simulink model "test_cost_function_only_without_delays"  (R2022a)
settings: Solver=FixedStepDiscrete  StartTime=0.0  StopTime=10.0  RelTol=1e-3
undefined symbols (not defined in the file or in its folder): f_c
libraries: hdlsllib x1
settings Model: DataTypeOverride=Off  Creator=Andre Merx  LastModifiedBy=Andre Merx
settings SolverCC: AlgebraicLoopSolver=TrustRegion
settings DataIOCC: LimitDataPoints=on  SaveOutput=off  SaveTime=off
settings OptimizationCC: BlockReduction=off  ConditionallyExecuteInputs=off  DefaultParameterBehavior=Inlined  LifeSpan=inf
settings DebuggingCC: AlgebraicLoopMsg=error  SingleTaskRateTransMsg=error  UnconnectedInputMsg=warning  UnconnectedOutputMsg=warning  UnconnectedLineMsg=warning  AllowSymbolicDim=off  StrictBusMsg=ErrorOnBusTreatedAsVector  SFUnexpectedBacktrackingDiag=warning  SFNoUnconditionalDefaultTransitionDiag=warning  SFExecutionAtInitializationDiag=none  SFMachineParentedDataDiag=warning  ArithmeticOperatorsInVariantConditions=warning
settings HardwareCC: ProdBitPerPointer=32  ProdBitPerSizeT=32  ProdBitPerPtrDiffT=32  ProdLargestAtomicFloat=None  ProdIntDivRoundTo=Undefined  ProdEndianess=Unspecified  ProdWordSize=32  ProdHWDeviceType=ASIC/FPGA->ASIC/FPGA  ProdEqTarget=off
settings SFSimCC: SimUseLocalCustomCode=off  CustomCodeUndefinedFunction=UseInterfaceOnly
settings RTWCC: RTWUseLocalCustomCode=off
settings CodeAppCC: StateflowObjectComments=on
settings GRTTargetCC: TargetLangStandard=C89/C90 (ANSI)
settings ConfigComp: CovScope=ReferencedModels  CovMetricSettings=dw  CovSaveCumulativeToWorkspaceVar=on  CovSaveSingleToWorkspaceVar=on  CovExternalEMLEnable=off  CovSFcnEnable=off

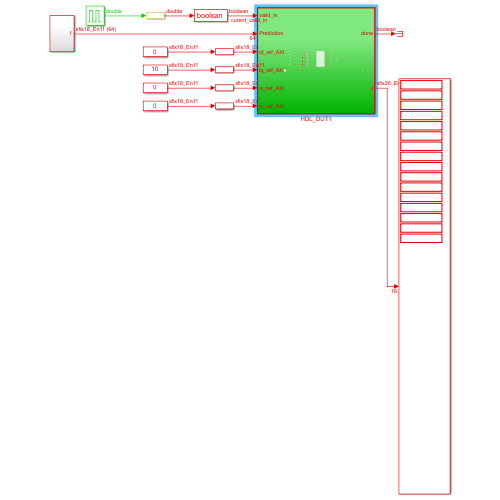
[thumbnail: Simulink's stored preview of the top-level diagram]
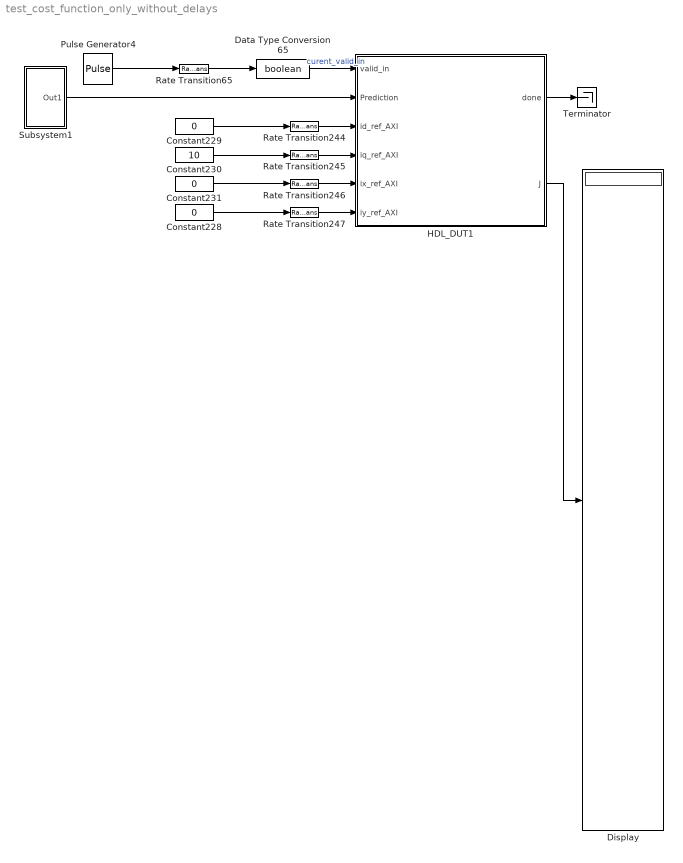
== system test_cost_function_only_without_delays ==
  Constant228 : Constant  Value=0  OutDataTypeStr=fixdt(1,18,11)  SampleTime=-1
  Constant229 : Constant  Value=0  OutDataTypeStr=fixdt(1,18,11)  SampleTime=-1
  Constant230 : Constant  Value=10  OutDataTypeStr=fixdt(1,18,11)  SampleTime=-1
  Constant231 : Constant  Value=0  OutDataTypeStr=fixdt(1,18,11)  SampleTime=-1
  Data Type Conversion65 : DataTypeConversion  OutDataTypeStr=boolean  SaturateOnIntegerOverflow=off  RndMeth=Floor
  Display : Display
  HDL_DUT1 : Subsystem  TreatAsAtomicUnit=on
  Pulse Generator4 : DiscretePulseGenerator  PulseType=Time based  Period=1/f_c
  Rate Transition{65,244..247} (5 alike) : RateTransition  OutPortSampleTime=Rt
  Subsystem1 : Subsystem
  Terminator : Terminator
  wires:
  Constant228/1 -> Rate Transition247/1
  Constant231/1 -> Rate Transition246/1
  Rate Transition247/1 -> HDL_DUT1/6(iy_ref_AXI)
  Rate Transition245/1 -> HDL_DUT1/4(iq_ref_AXI)
  Subsystem1/1(Out1) -> HDL_DUT1/2(Prediction)
  Constant229/1 -> Rate Transition244/1
  Constant230/1 -> Rate Transition245/1
  Rate Transition246/1 -> HDL_DUT1/5(ix_ref_AXI)
  Rate Transition244/1 -> HDL_DUT1/3(id_ref_AXI)
  Pulse Generator4/1 -> Rate Transition65/1
  Rate Transition65/1 -> Data Type Conversion65/1
  Data Type Conversion65/1 -> HDL_DUT1/1(valid_in)  "curent_valid_in"
  HDL_DUT1/1(done) -> Terminator/1
  HDL_DUT1/2(J) -> Display/1

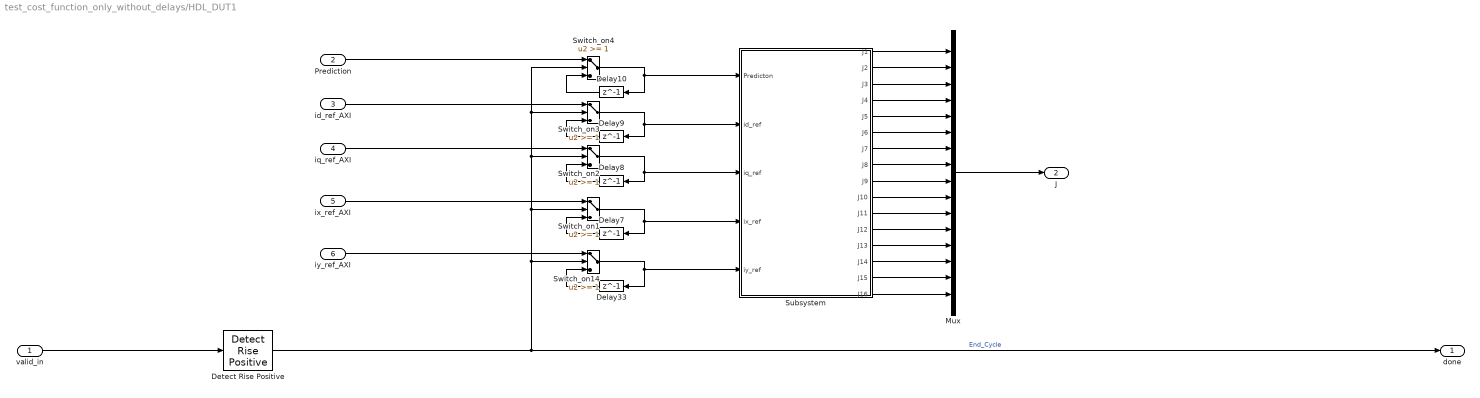
== system test_cost_function_only_without_delays/HDL_DUT1 ==
  valid_in : Inport
  Prediction : Inport  Port=2
  id_ref_AXI : Inport  Port=3
  iq_ref_AXI : Inport  Port=4
  ix_ref_AXI : Inport  Port=5
  iy_ref_AXI : Inport  Port=6
  Delay{7..10,33} (5 alike) : Delay  DelayLength=1
  Detect Rise Positive : hdlsllib/Logic and Bit Operations/Detect Rise Positive  vinit=0  OutDataTypeStr=boolean
      settings: SourceProductBaseCode=SL
  Mux : Mux  Inputs=16
  Subsystem : Subsystem
  Switch_on{1..4,14} (5 alike) : Switch  Threshold=1  OutDataTypeStr=fixdt(1,18,11)  RndMeth=Simplest  SaturateOnIntegerOverflow=off  InputSameDT=off
  done : Outport
  J : Outport  Port=2
  wires:
  iy_ref_AXI/1 -> Switch_on14/1
  Switch_on14/1 -> Delay33/1, Subsystem/5(iy_ref)
  Delay33/1 -> Switch_on14/3
  Delay7/1 -> Switch_on1/3
  ix_ref_AXI/1 -> Switch_on1/1
  Switch_on1/1 -> Subsystem/4(ix_ref), Delay7/1
  Delay8/1 -> Switch_on2/3
  iq_ref_AXI/1 -> Switch_on2/1
  Switch_on2/1 -> Subsystem/3(iq_ref), Delay8/1
  Delay9/1 -> Switch_on3/3
  id_ref_AXI/1 -> Switch_on3/1
  Switch_on3/1 -> Subsystem/2(id_ref), Delay9/1
  Delay10/1 -> Switch_on4/3
  Detect Rise Positive/1 -> done/1, Switch_on4/2, Switch_on3/2, Switch_on2/2, Switch_on1/2, Switch_on14/2  "End_Cycle"
  Prediction/1 -> Switch_on4/1
  Switch_on4/1 -> Delay10/1, Subsystem/1(Predicton)
  Subsystem/1(J1) -> Mux/1
  Subsystem/2(J2) -> Mux/2
  Subsystem/3(J3) -> Mux/3
  Subsystem/4(J4) -> Mux/4
  Subsystem/5(J5) -> Mux/5
  Subsystem/6(J6) -> Mux/6
  Subsystem/7(J7) -> Mux/7
  Subsystem/8(J8) -> Mux/8
  Subsystem/9(J9) -> Mux/9
  Subsystem/10(J10) -> Mux/10
  Subsystem/11(J11) -> Mux/11
  Subsystem/12(J12) -> Mux/12
  Subsystem/13(J13) -> Mux/13
  Subsystem/14(J14) -> Mux/14
  Subsystem/15(J15) -> Mux/15
  Subsystem/16(J16) -> Mux/16
  Mux/1 -> J/1
  valid_in/1 -> Detect Rise Positive/1

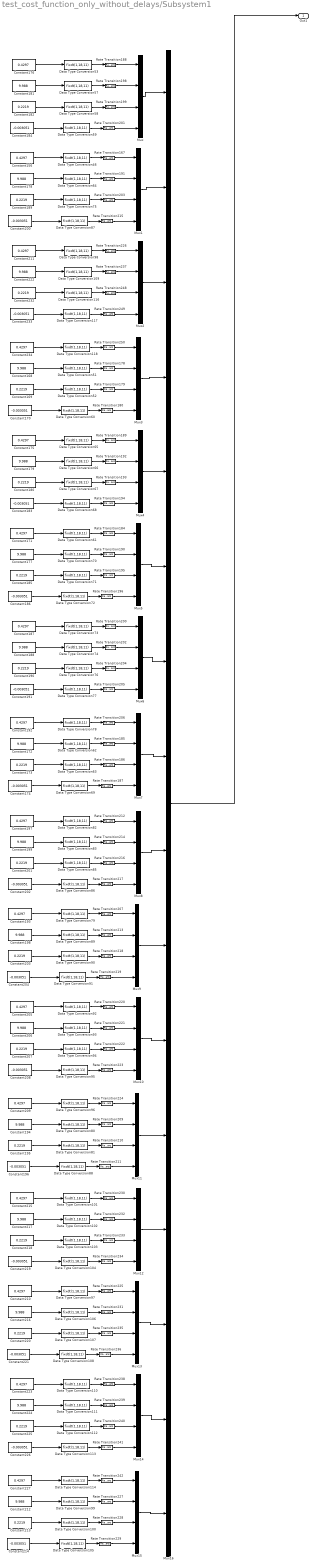
== system test_cost_function_only_without_delays/Subsystem1 ==
  Constant{156,171,175..176,187,192..193,197,205,209..211,215,223,227,234} (16 alike) : Constant  Value=0.4297
  Constant{168,172,177..179,181,188,194,198..199,206,212,216..217,222,224} (16 alike) : Constant  Value=9.988
  Constant{169,173,180,182,185,189..190,195,201,203,207,213,218,220,225,232} (16 alike) : Constant  Value=0.2219
  Constant{170,174,183..184,186,191,196,200,202,204,208,214,219,221,226,233} (16 alike) : Constant  Value=-0.003051
  Data Type Conversion{46,51..53,57..83,85..114,116..118} (64 alike) : DataTypeConversion  OutDataTypeStr=fixdt(1,18,11)  SaturateOnIntegerOverflow=off  RndMeth=Floor
  Mux{,1..15} (16 alike) : Mux
  Mux16 : Mux  Inputs=16
  Rate Transition{167,178..180,184..196,198..207,209..242,248..250} (64 alike) : RateTransition  OutPortSampleTime=Rt
  Out1 : Outport
  wires:
  Constant220/1 -> Data Type Conversion107/1
  Constant205/1 -> Data Type Conversion92/1
  Rate Transition215/1 -> Mux1/4
  Data Type Conversion69/1 -> Rate Transition187/1
  Data Type Conversion71/1 -> Rate Transition195/1
  Data Type Conversion117/1 -> Rate Transition249/1
  Data Type Conversion87/1 -> Rate Transition215/1
  Constant193/1 -> Data Type Conversion79/1
  Constant182/1 -> Data Type Conversion58/1
  Mux13/1 -> Mux16/14
  Data Type Conversion88/1 -> Rate Transition211/1
  Rate Transition202/1 -> Mux6/2
  Data Type Conversion70/1 -> Rate Transition190/1
  Constant169/1 -> Data Type Conversion52/1
  Rate Transition178/1 -> Mux3/2
  Constant175/1 -> Data Type Conversion65/1
  Rate Transition193/1 -> Mux4/3
  Data Type Conversion63/1 -> Rate Transition186/1
  Data Type Conversion72/1 -> Rate Transition196/1
  Data Type Conversion83/1 -> Rate Transition214/1
  Data Type Conversion75/1 -> Rate Transition203/1
  Rate Transition201/1 -> Mux/4
  Mux7/1 -> Mux16/8
  Rate Transition184/1 -> Mux5/1
  Data Type Conversion79/1 -> Rate Transition207/1
  Data Type Conversion65/1 -> Rate Transition189/1
  Data Type Conversion66/1 -> Rate Transition192/1
  Rate Transition190/1 -> Mux5/2
  Rate Transition196/1 -> Mux5/4
  Constant168/1 -> Data Type Conversion51/1
  Constant183/1 -> Data Type Conversion68/1
  Rate Transition187/1 -> Mux7/4
  Rate Transition222/1 -> Mux10/3
  Constant188/1 -> Data Type Conversion74/1
  Rate Transition189/1 -> Mux4/1
  Constant195/1 -> Data Type Conversion81/1
  Constant214/1 -> Data Type Conversion105/1
  Mux/1 -> Mux16/1
  Rate Transition224/1 -> Mux11/1
  Constant172/1 -> Data Type Conversion62/1
  Rate Transition232/1 -> Mux12/2
  Constant202/1 -> Data Type Conversion86/1
  Data Type Conversion61/1 -> Rate Transition184/1
  Data Type Conversion93/1 -> Rate Transition221/1
  Data Type Conversion64/1 -> Rate Transition191/1
  Rate Transition227/1 -> Mux15/2
  Constant187/1 -> Data Type Conversion73/1
  Constant199/1 -> Data Type Conversion83/1
  Data Type Conversion74/1 -> Rate Transition202/1
  Rate Transition192/1 -> Mux4/2
  Rate Transition210/1 -> Mux11/3
  Data Type Conversion108/1 -> Rate Transition236/1
  Constant208/1 -> Data Type Conversion95/1
  Constant170/1 -> Data Type Conversion60/1
  Data Type Conversion86/1 -> Rate Transition217/1
  Rate Transition238/1 -> Mux14/1
  Data Type Conversion116/1 -> Rate Transition248/1
  Mux8/1 -> Mux16/9
  Constant176/1 -> Data Type Conversion53/1
  Rate Transition200/1 -> Mux6/1
  Rate Transition230/1 -> Mux12/1
  Rate Transition250/1 -> Mux3/1
  Data Type Conversion102/1 -> Rate Transition232/1
  Constant222/1 -> Data Type Conversion109/1
  Constant184/1 -> Data Type Conversion59/1
  Constant179/1 -> Data Type Conversion66/1
  Constant221/1 -> Data Type Conversion108/1
  Mux16/1 -> Out1/1
  Data Type Conversion118/1 -> Rate Transition250/1
  Data Type Conversion80/1 -> Rate Transition209/1
  Constant215/1 -> Data Type Conversion101/1
  Data Type Conversion53/1 -> Rate Transition188/1
  Rate Transition194/1 -> Mux4/4
  Constant180/1 -> Data Type Conversion67/1
  Rate Transition217/1 -> Mux8/4
  Data Type Conversion100/1 -> Rate Transition228/1
  Constant233/1 -> Data Type Conversion117/1
  Rate Transition167/1 -> Mux1/1
  Constant196/1 -> Data Type Conversion88/1
  Constant211/1 -> Data Type Conversion98/1
  Data Type Conversion67/1 -> Rate Transition193/1
  Rate Transition199/1 -> Mux/3
  Rate Transition186/1 -> Mux7/3
  Rate Transition188/1 -> Mux/1
  Constant209/1 -> Data Type Conversion96/1
  Constant232/1 -> Data Type Conversion116/1
  Mux15/1 -> Mux16/16
  Rate Transition226/1 -> Mux2/1
  Rate Transition211/1 -> Mux11/4
  Data Type Conversion57/1 -> Rate Transition198/1
  Rate Transition237/1 -> Mux2/2
  Constant156/1 -> Data Type Conversion46/1
  Constant181/1 -> Data Type Conversion57/1
  Rate Transition248/1 -> Mux2/3
  Data Type Conversion101/1 -> Rate Transition230/1
  Data Type Conversion73/1 -> Rate Transition200/1
  Data Type Conversion60/1 -> Rate Transition180/1
  Constant178/1 -> Data Type Conversion64/1
  Constant201/1 -> Data Type Conversion85/1
  Constant173/1 -> Data Type Conversion63/1
  Mux10/1 -> Mux16/11
  Rate Transition203/1 -> Mux1/3
  Constant177/1 -> Data Type Conversion70/1
  Data Type Conversion114/1 -> Rate Transition242/1
  Data Type Conversion109/1 -> Rate Transition237/1
  Constant174/1 -> Data Type Conversion69/1
  Rate Transition235/1 -> Mux13/3
  Constant225/1 -> Data Type Conversion112/1
  Constant185/1 -> Data Type Conversion71/1
  Constant194/1 -> Data Type Conversion80/1
  Data Type Conversion59/1 -> Rate Transition201/1
  Rate Transition198/1 -> Mux/2
  Constant223/1 -> Data Type Conversion110/1
  Rate Transition180/1 -> Mux3/4
  Constant190/1 -> Data Type Conversion76/1
  Constant206/1 -> Data Type Conversion93/1
  Data Type Conversion78/1 -> Rate Transition206/1
  Rate Transition195/1 -> Mux5/3
  Data Type Conversion112/1 -> Rate Transition240/1
  Constant186/1 -> Data Type Conversion72/1
  Data Type Conversion62/1 -> Rate Transition185/1
  Constant210/1 -> Data Type Conversion97/1
  Constant224/1 -> Data Type Conversion111/1
  Data Type Conversion107/1 -> Rate Transition235/1
  Rate Transition249/1 -> Mux2/4
  Rate Transition236/1 -> Mux13/4
  Rate Transition242/1 -> Mux15/1
  Mux14/1 -> Mux16/15
  Rate Transition179/1 -> Mux3/3
  Data Type Conversion82/1 -> Rate Transition212/1
  Data Type Conversion111/1 -> Rate Transition239/1
  Rate Transition220/1 -> Mux10/1
  Constant227/1 -> Data Type Conversion114/1
  Mux12/1 -> Mux16/13
  Mux11/1 -> Mux16/12
  Data Type Conversion85/1 -> Rate Transition216/1
  Data Type Conversion104/1 -> Rate Transition234/1
  Data Type Conversion68/1 -> Rate Transition194/1
  Constant200/1 -> Data Type Conversion87/1
  Data Type Conversion46/1 -> Rate Transition167/1
  Rate Transition205/1 -> Mux6/4
  Data Type Conversion52/1 -> Rate Transition179/1
  Mux6/1 -> Mux16/7
  Constant212/1 -> Data Type Conversion99/1
  Constant204/1 -> Data Type Conversion91/1
  Constant219/1 -> Data Type Conversion104/1
  Data Type Conversion77/1 -> Rate Transition205/1
  Rate Transition209/1 -> Mux11/2
  Mux1/1 -> Mux16/2
  Data Type Conversion97/1 -> Rate Transition225/1
  Mux5/1 -> Mux16/6
  Data Type Conversion105/1 -> Rate Transition229/1
  Rate Transition228/1 -> Mux15/3
  Mux9/1 -> Mux16/10
  Mux2/1 -> Mux16/3
  Rate Transition218/1 -> Mux9/3
  Rate Transition239/1 -> Mux14/2
  Mux3/1 -> Mux16/4
  Rate Transition241/1 -> Mux14/4
  Rate Transition231/1 -> Mux13/2
  Data Type Conversion99/1 -> Rate Transition227/1
  Constant216/1 -> Data Type Conversion106/1
  Constant213/1 -> Data Type Conversion100/1
  Rate Transition240/1 -> Mux14/3
  Rate Transition229/1 -> Mux15/4
  Rate Transition234/1 -> Mux12/4
  Rate Transition207/1 -> Mux9/1
  Rate Transition225/1 -> Mux13/1
  Data Type Conversion106/1 -> Rate Transition231/1
  Constant234/1 -> Data Type Conversion118/1
  Constant171/1 -> Data Type Conversion61/1
  Mux4/1 -> Mux16/5
  Rate Transition219/1 -> Mux9/4
  Data Type Conversion98/1 -> Rate Transition226/1
  Constant217/1 -> Data Type Conversion102/1
  Constant192/1 -> Data Type Conversion78/1
  Constant226/1 -> Data Type Conversion113/1
  Data Type Conversion113/1 -> Rate Transition241/1
  Rate Transition204/1 -> Mux6/3
  Data Type Conversion58/1 -> Rate Transition199/1
  Constant191/1 -> Data Type Conversion77/1
  Rate Transition216/1 -> Mux8/3
  Rate Transition212/1 -> Mux8/1
  Data Type Conversion103/1 -> Rate Transition233/1
  Data Type Conversion110/1 -> Rate Transition238/1
  Data Type Conversion91/1 -> Rate Transition219/1
  Data Type Conversion94/1 -> Rate Transition222/1
  Constant218/1 -> Data Type Conversion103/1
  Constant198/1 -> Data Type Conversion89/1
  Rate Transition213/1 -> Mux9/2
  Data Type Conversion96/1 -> Rate Transition224/1
  Constant203/1 -> Data Type Conversion90/1
  Data Type Conversion76/1 -> Rate Transition204/1
  Rate Transition233/1 -> Mux12/3
  Rate Transition191/1 -> Mux1/2
  Constant189/1 -> Data Type Conversion75/1
  Data Type Conversion81/1 -> Rate Transition210/1
  Rate Transition185/1 -> Mux7/2
  Data Type Conversion89/1 -> Rate Transition213/1
  Data Type Conversion51/1 -> Rate Transition178/1
  Rate Transition221/1 -> Mux10/2
  Constant207/1 -> Data Type Conversion94/1
  Data Type Conversion95/1 -> Rate Transition223/1
  Rate Transition206/1 -> Mux7/1
  Rate Transition214/1 -> Mux8/2
  Constant197/1 -> Data Type Conversion82/1
  Data Type Conversion92/1 -> Rate Transition220/1
  Rate Transition223/1 -> Mux10/4
  Data Type Conversion90/1 -> Rate Transition218/1

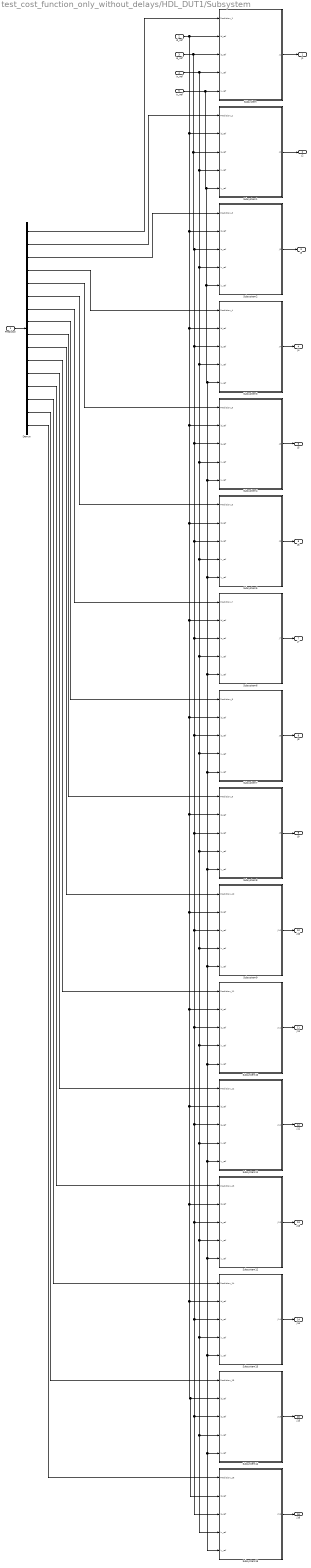
== system test_cost_function_only_without_delays/HDL_DUT1/Subsystem ==
  Predicton : Inport
  id_ref : Inport  Port=2
  iq_ref : Inport  Port=3
  ix_ref : Inport  Port=4
  iy_ref : Inport  Port=5
  Demux : Demux  Outputs=16
  Subsystem : Subsystem
  Subsystem1 : Subsystem
  Subsystem10 : Subsystem
  Subsystem11 : Subsystem
  Subsystem12 : Subsystem
  Subsystem13 : Subsystem
  Subsystem14 : Subsystem
  Subsystem15 : Subsystem
  Subsystem2 : Subsystem
  Subsystem3 : Subsystem
  Subsystem4 : Subsystem
  Subsystem5 : Subsystem
  Subsystem6 : Subsystem
  Subsystem7 : Subsystem
  Subsystem8 : Subsystem
  Subsystem9 : Subsystem
  J1 : Outport
  J2 : Outport  Port=2
  J3 : Outport  Port=3
  J4 : Outport  Port=4
  J5 : Outport  Port=5
  J6 : Outport  Port=6
  J7 : Outport  Port=7
  J8 : Outport  Port=8
  J9 : Outport  Port=9
  J10 : Outport  Port=10
  J11 : Outport  Port=11
  J12 : Outport  Port=12
  J13 : Outport  Port=13
  J14 : Outport  Port=14
  J15 : Outport  Port=15
  J16 : Outport  Port=16
  wires:
  Predicton/1 -> Demux/1
  iy_ref/1 -> Subsystem/5(iy_ref), Subsystem15/5(iy_ref), Subsystem14/5(iy_ref), Subsystem13/5(iy_ref), Subsystem12/5(iy_ref), Subsystem11/5(iy_ref), Subsystem10/5(iy_ref), Subsystem9/5(iy_ref), Subsystem8/5(iy_ref), Subsystem7/5(iy_ref), Subsystem6/5(iy_ref), Subsystem5/5(iy_ref), Subsystem4/5(iy_ref), Subsystem3/5(iy_ref), Subsystem2/5(iy_ref), Subsystem1/5(iy_ref)
  ix_ref/1 -> Subsystem/4(ix_ref), Subsystem15/4(ix_ref), Subsystem14/4(ix_ref), Subsystem13/4(ix_ref), Subsystem12/4(ix_ref), Subsystem11/4(ix_ref), Subsystem10/4(ix_ref), Subsystem9/4(ix_ref), Subsystem8/4(ix_ref), Subsystem7/4(ix_ref), Subsystem6/4(ix_ref), Subsystem5/4(ix_ref), Subsystem4/4(ix_ref), Subsystem3/4(ix_ref), Subsystem2/4(ix_ref), Subsystem1/4(ix_ref)
  iq_ref/1 -> Subsystem/3(iq_ref), Subsystem15/3(iq_ref), Subsystem14/3(iq_ref), Subsystem13/3(iq_ref), Subsystem12/3(iq_ref), Subsystem11/3(iq_ref), Subsystem10/3(iq_ref), Subsystem9/3(iq_ref), Subsystem8/3(iq_ref), Subsystem7/3(iq_ref), Subsystem6/3(iq_ref), Subsystem5/3(iq_ref), Subsystem4/3(iq_ref), Subsystem3/3(iq_ref), Subsystem2/3(iq_ref), Subsystem1/3(iq_ref)
  id_ref/1 -> Subsystem15/2(id_ref), Subsystem14/2(id_ref), Subsystem13/2(id_ref), Subsystem12/2(id_ref), Subsystem11/2(id_ref), Subsystem10/2(id_ref), Subsystem9/2(id_ref), Subsystem8/2(id_ref), Subsystem7/2(id_ref), Subsystem6/2(id_ref), Subsystem5/2(id_ref), Subsystem4/2(id_ref), Subsystem3/2(id_ref), Subsystem2/2(id_ref), Subsystem1/2(id_ref), Subsystem/2(id_ref)
  Demux/1 -> Subsystem/1(Prediction_1)
  Demux/2 -> Subsystem1/1(Prediction_2)
  Demux/3 -> Subsystem2/1(Prediction_3)
  Demux/4 -> Subsystem3/1(Prediction_4)
  Demux/5 -> Subsystem4/1(Prediction_5)
  Demux/6 -> Subsystem5/1(Prediction_6)
  Demux/7 -> Subsystem6/1(Prediction_7)
  Demux/8 -> Subsystem7/1(Prediction_8)
  Demux/9 -> Subsystem8/1(Prediction_9)
  Demux/10 -> Subsystem9/1(Prediction_10)
  Demux/11 -> Subsystem10/1(Prediction_11)
  Demux/12 -> Subsystem11/1(Prediction_12)
  Demux/13 -> Subsystem12/1(Prediction_13)
  Demux/14 -> Subsystem13/1(Prediction_14)
  Demux/15 -> Subsystem14/1(Prediction_15)
  Demux/16 -> Subsystem15/1(Prediction_16)
  Subsystem/1(J1) -> J1/1
  Subsystem1/1(J2) -> J2/1
  Subsystem2/1(J3) -> J3/1
  Subsystem3/1(J4) -> J4/1
  Subsystem4/1(J5) -> J5/1
  Subsystem5/1(J6) -> J6/1
  Subsystem6/1(J7) -> J7/1
  Subsystem7/1(J8) -> J8/1
  Subsystem8/1(J9) -> J9/1
  Subsystem9/1(J10) -> J10/1
  Subsystem10/1(J11) -> J11/1
  Subsystem11/1(J12) -> J12/1
  Subsystem12/1(J13) -> J13/1
  Subsystem13/1(J14) -> J14/1
  Subsystem14/1(J15) -> J15/1
  Subsystem15/1(J16) -> J16/1

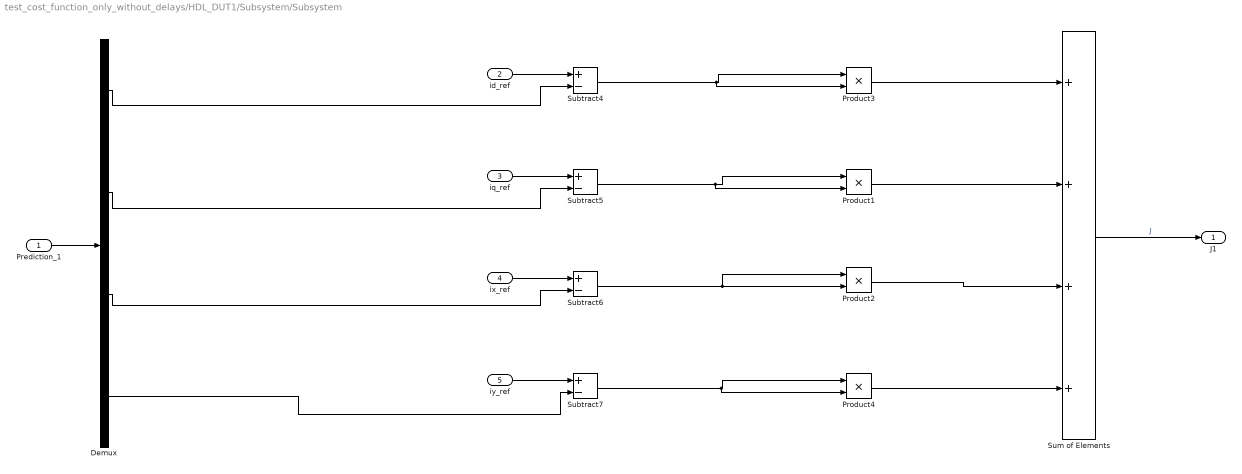
== system test_cost_function_only_without_delays/HDL_DUT1/Subsystem/Subsystem ==
  Prediction_1 : Inport
  id_ref : Inport  Port=2
  iq_ref : Inport  Port=3
  ix_ref : Inport  Port=4
  iy_ref : Inport  Port=5
  Demux : Demux
  Product{1..4} (4 alike) : Product  OutDataTypeStr=fixdt(1,20,11)
  Subtract{4..7} (4 alike) : Sum  Inputs=+-  OutDataTypeStr=fixdt(1,20,11)
  Sum of Elements : Sum  Inputs=++++  OutDataTypeStr=fixdt(1,20,11)
  J1 : Outport
  wires:
  Prediction_1/1 -> Demux/1
  iy_ref/1 -> Subtract7/1
  Demux/3 -> Subtract6/2
  Sum of Elements/1 -> J1/1  "J"
  iq_ref/1 -> Subtract5/1
  id_ref/1 -> Subtract4/1
  Demux/2 -> Subtract5/2
  ix_ref/1 -> Subtract6/1
  Demux/4 -> Subtract7/2
  Demux/1 -> Subtract4/2
  Product3/1 -> Sum of Elements/1
  Product1/1 -> Sum of Elements/2
  Product2/1 -> Sum of Elements/3
  Product4/1 -> Sum of Elements/4
  Subtract4/1 -> Product3/2, Product3/1
  Subtract5/1 -> Product1/2, Product1/1
  Subtract6/1 -> Product2/2, Product2/1
  Subtract7/1 -> Product4/2, Product4/1

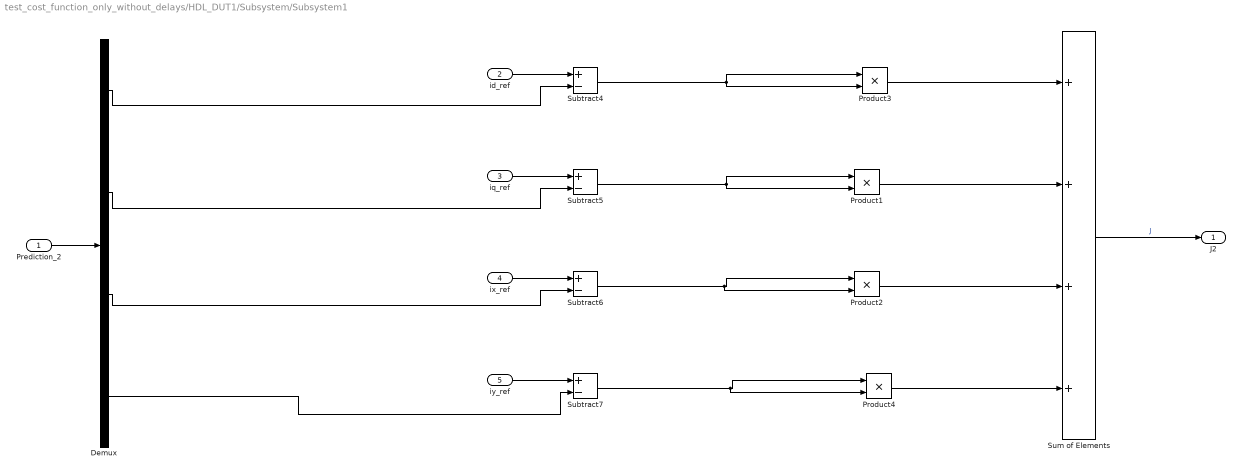
== system test_cost_function_only_without_delays/HDL_DUT1/Subsystem/Subsystem1 ==
  Prediction_2 : Inport
  id_ref : Inport  Port=2
  iq_ref : Inport  Port=3
  ix_ref : Inport  Port=4
  iy_ref : Inport  Port=5
  Demux : Demux
  Product{1..4} (4 alike) : Product  OutDataTypeStr=fixdt(1,20,11)
  Subtract{4..7} (4 alike) : Sum  Inputs=+-  OutDataTypeStr=fixdt(1,20,11)
  Sum of Elements : Sum  Inputs=++++  OutDataTypeStr=fixdt(1,20,11)
  J2 : Outport
  wires:
  Prediction_2/1 -> Demux/1
  iy_ref/1 -> Subtract7/1
  Demux/3 -> Subtract6/2
  Sum of Elements/1 -> J2/1  "J"
  iq_ref/1 -> Subtract5/1
  id_ref/1 -> Subtract4/1
  Demux/2 -> Subtract5/2
  ix_ref/1 -> Subtract6/1
  Demux/4 -> Subtract7/2
  Demux/1 -> Subtract4/2
  Product3/1 -> Sum of Elements/1
  Product1/1 -> Sum of Elements/2
  Product2/1 -> Sum of Elements/3
  Product4/1 -> Sum of Elements/4
  Subtract4/1 -> Product3/2, Product3/1
  Subtract5/1 -> Product1/2, Product1/1
  Subtract6/1 -> Product2/2, Product2/1
  Subtract7/1 -> Product4/2, Product4/1

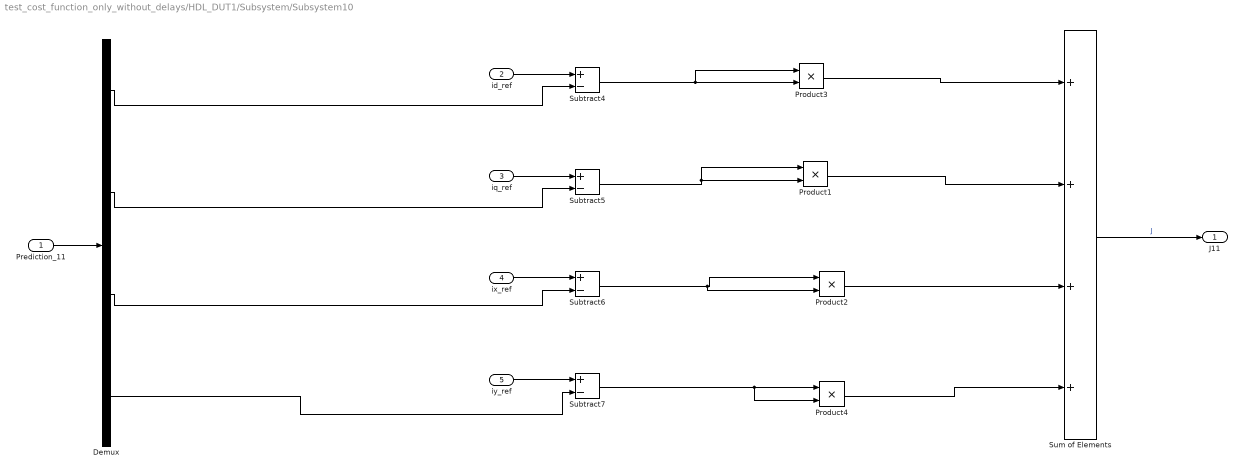
== system test_cost_function_only_without_delays/HDL_DUT1/Subsystem/Subsystem10 ==
  Prediction_11 : Inport
  id_ref : Inport  Port=2
  iq_ref : Inport  Port=3
  ix_ref : Inport  Port=4
  iy_ref : Inport  Port=5
  Demux : Demux
  Product{1..4} (4 alike) : Product  OutDataTypeStr=fixdt(1,20,11)
  Subtract{4..7} (4 alike) : Sum  Inputs=+-  OutDataTypeStr=fixdt(1,20,11)
  Sum of Elements : Sum  Inputs=++++  OutDataTypeStr=fixdt(1,20,11)
  J11 : Outport
  wires:
  Prediction_11/1 -> Demux/1
  iy_ref/1 -> Subtract7/1
  Demux/3 -> Subtract6/2
  Sum of Elements/1 -> J11/1  "J"
  iq_ref/1 -> Subtract5/1
  id_ref/1 -> Subtract4/1
  Demux/2 -> Subtract5/2
  ix_ref/1 -> Subtract6/1
  Demux/4 -> Subtract7/2
  Demux/1 -> Subtract4/2
  Product3/1 -> Sum of Elements/1
  Product1/1 -> Sum of Elements/2
  Product2/1 -> Sum of Elements/3
  Product4/1 -> Sum of Elements/4
  Subtract4/1 -> Product3/2, Product3/1
  Subtract5/1 -> Product1/2, Product1/1
  Subtract6/1 -> Product2/2, Product2/1
  Subtract7/1 -> Product4/2, Product4/1

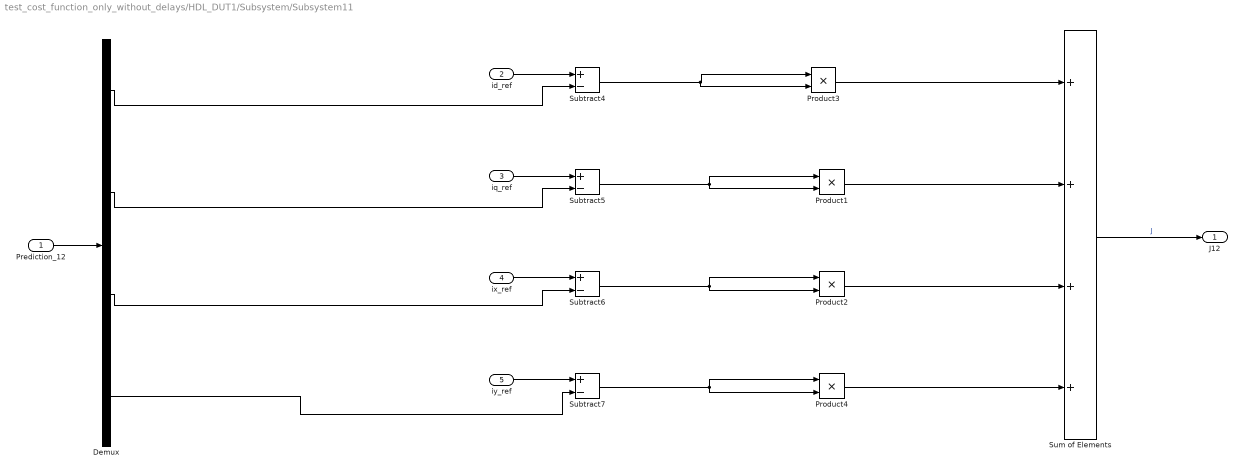
== system test_cost_function_only_without_delays/HDL_DUT1/Subsystem/Subsystem11 ==
  Prediction_12 : Inport
  id_ref : Inport  Port=2
  iq_ref : Inport  Port=3
  ix_ref : Inport  Port=4
  iy_ref : Inport  Port=5
  Demux : Demux
  Product{1..4} (4 alike) : Product  OutDataTypeStr=fixdt(1,20,11)
  Subtract{4..7} (4 alike) : Sum  Inputs=+-  OutDataTypeStr=fixdt(1,20,11)
  Sum of Elements : Sum  Inputs=++++  OutDataTypeStr=fixdt(1,20,11)
  J12 : Outport
  wires:
  Prediction_12/1 -> Demux/1
  iy_ref/1 -> Subtract7/1
  Demux/3 -> Subtract6/2
  Sum of Elements/1 -> J12/1  "J"
  iq_ref/1 -> Subtract5/1
  id_ref/1 -> Subtract4/1
  Demux/2 -> Subtract5/2
  ix_ref/1 -> Subtract6/1
  Demux/4 -> Subtract7/2
  Demux/1 -> Subtract4/2
  Product3/1 -> Sum of Elements/1
  Product1/1 -> Sum of Elements/2
  Product2/1 -> Sum of Elements/3
  Product4/1 -> Sum of Elements/4
  Subtract4/1 -> Product3/2, Product3/1
  Subtract5/1 -> Product1/1, Product1/2
  Subtract6/1 -> Product2/2, Product2/1
  Subtract7/1 -> Product4/2, Product4/1

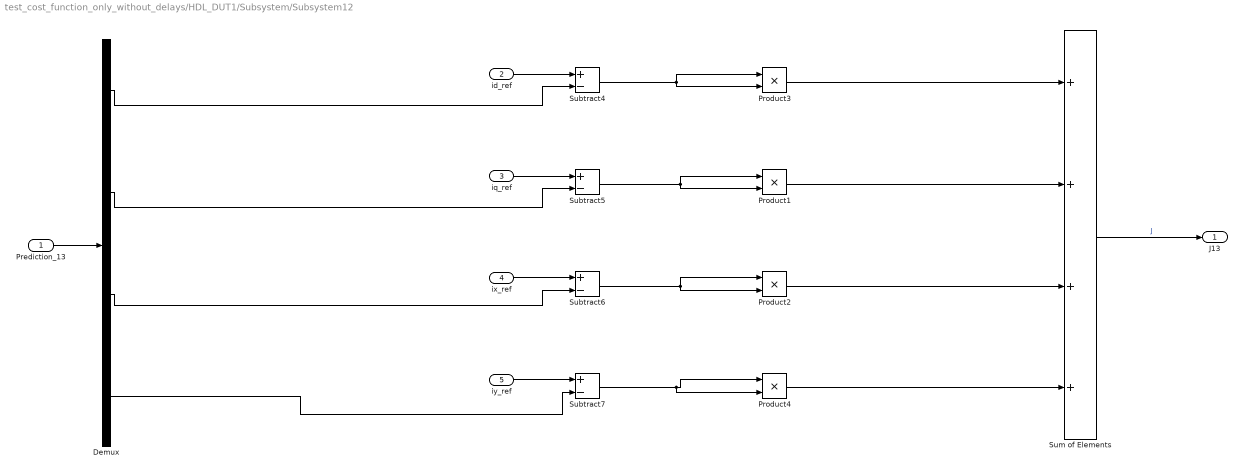
== system test_cost_function_only_without_delays/HDL_DUT1/Subsystem/Subsystem12 ==
  Prediction_13 : Inport
  id_ref : Inport  Port=2
  iq_ref : Inport  Port=3
  ix_ref : Inport  Port=4
  iy_ref : Inport  Port=5
  Demux : Demux
  Product{1..4} (4 alike) : Product  OutDataTypeStr=fixdt(1,20,11)
  Subtract{4..7} (4 alike) : Sum  Inputs=+-  OutDataTypeStr=fixdt(1,20,11)
  Sum of Elements : Sum  Inputs=++++  OutDataTypeStr=fixdt(1,20,11)
  J13 : Outport
  wires:
  Prediction_13/1 -> Demux/1
  iy_ref/1 -> Subtract7/1
  Demux/3 -> Subtract6/2
  Sum of Elements/1 -> J13/1  "J"
  iq_ref/1 -> Subtract5/1
  id_ref/1 -> Subtract4/1
  Demux/2 -> Subtract5/2
  ix_ref/1 -> Subtract6/1
  Demux/4 -> Subtract7/2
  Demux/1 -> Subtract4/2
  Product3/1 -> Sum of Elements/1
  Product1/1 -> Sum of Elements/2
  Product2/1 -> Sum of Elements/3
  Product4/1 -> Sum of Elements/4
  Subtract4/1 -> Product3/2, Product3/1
  Subtract5/1 -> Product1/2, Product1/1
  Subtract6/1 -> Product2/2, Product2/1
  Subtract7/1 -> Product4/2, Product4/1

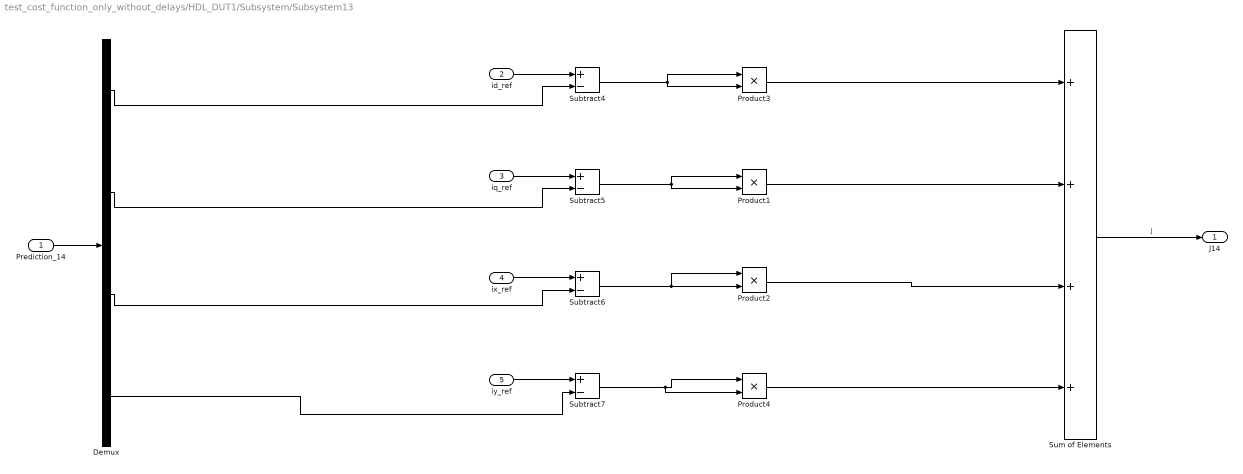
== system test_cost_function_only_without_delays/HDL_DUT1/Subsystem/Subsystem13 ==
  Prediction_14 : Inport
  id_ref : Inport  Port=2
  iq_ref : Inport  Port=3
  ix_ref : Inport  Port=4
  iy_ref : Inport  Port=5
  Demux : Demux
  Product{1..4} (4 alike) : Product  OutDataTypeStr=fixdt(1,20,11)
  Subtract{4..7} (4 alike) : Sum  Inputs=+-  OutDataTypeStr=fixdt(1,20,11)
  Sum of Elements : Sum  Inputs=++++  OutDataTypeStr=fixdt(1,20,11)
  J14 : Outport
  wires:
  Prediction_14/1 -> Demux/1
  iy_ref/1 -> Subtract7/1
  Demux/3 -> Subtract6/2
  Sum of Elements/1 -> J14/1  "J"
  iq_ref/1 -> Subtract5/1
  id_ref/1 -> Subtract4/1
  Demux/2 -> Subtract5/2
  ix_ref/1 -> Subtract6/1
  Demux/4 -> Subtract7/2
  Demux/1 -> Subtract4/2
  Product3/1 -> Sum of Elements/1
  Product1/1 -> Sum of Elements/2
  Product2/1 -> Sum of Elements/3
  Product4/1 -> Sum of Elements/4
  Subtract4/1 -> Product3/2, Product3/1
  Subtract5/1 -> Product1/1, Product1/2
  Subtract6/1 -> Product2/2, Product2/1
  Subtract7/1 -> Product4/2, Product4/1

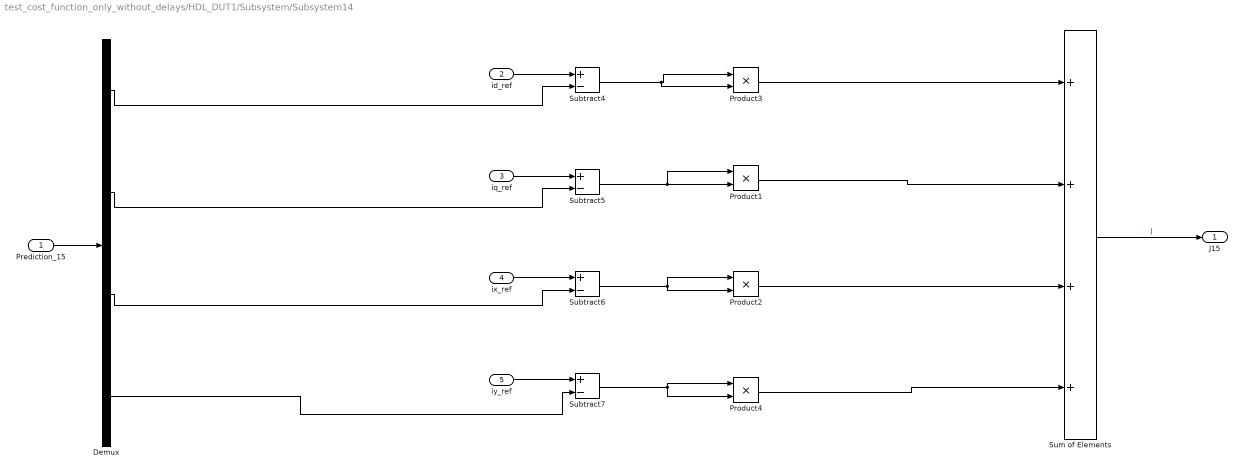
== system test_cost_function_only_without_delays/HDL_DUT1/Subsystem/Subsystem14 ==
  Prediction_15 : Inport
  id_ref : Inport  Port=2
  iq_ref : Inport  Port=3
  ix_ref : Inport  Port=4
  iy_ref : Inport  Port=5
  Demux : Demux
  Product{1..4} (4 alike) : Product  OutDataTypeStr=fixdt(1,20,11)
  Subtract{4..7} (4 alike) : Sum  Inputs=+-  OutDataTypeStr=fixdt(1,20,11)
  Sum of Elements : Sum  Inputs=++++  OutDataTypeStr=fixdt(1,20,11)
  J15 : Outport
  wires:
  Prediction_15/1 -> Demux/1
  iy_ref/1 -> Subtract7/1
  Demux/3 -> Subtract6/2
  Sum of Elements/1 -> J15/1  "J"
  iq_ref/1 -> Subtract5/1
  id_ref/1 -> Subtract4/1
  Demux/2 -> Subtract5/2
  ix_ref/1 -> Subtract6/1
  Demux/4 -> Subtract7/2
  Demux/1 -> Subtract4/2
  Product3/1 -> Sum of Elements/1
  Product1/1 -> Sum of Elements/2
  Product2/1 -> Sum of Elements/3
  Product4/1 -> Sum of Elements/4
  Subtract4/1 -> Product3/2, Product3/1
  Subtract5/1 -> Product1/1, Product1/2
  Subtract6/1 -> Product2/2, Product2/1
  Subtract7/1 -> Product4/2, Product4/1

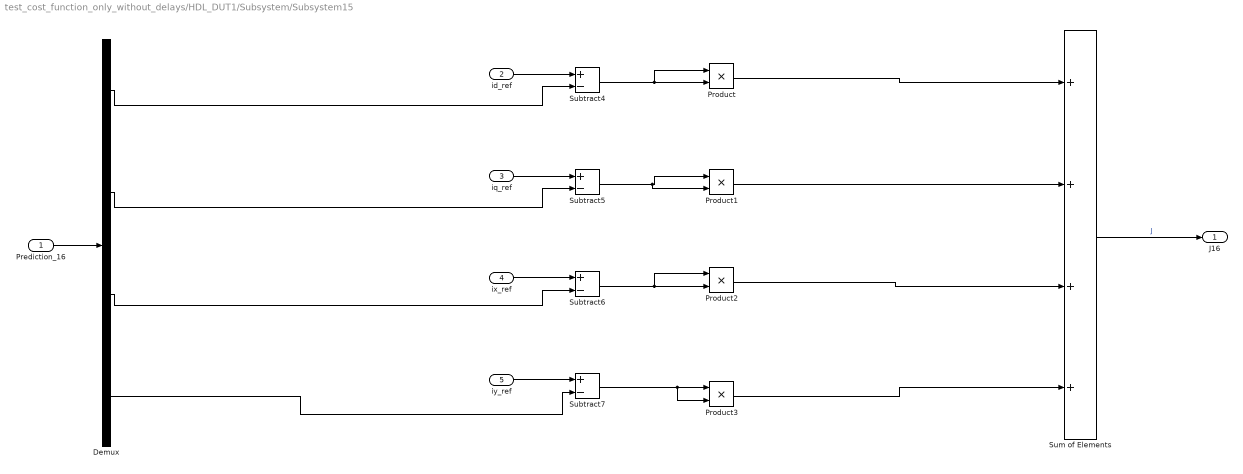
== system test_cost_function_only_without_delays/HDL_DUT1/Subsystem/Subsystem15 ==
  Prediction_16 : Inport
  id_ref : Inport  Port=2
  iq_ref : Inport  Port=3
  ix_ref : Inport  Port=4
  iy_ref : Inport  Port=5
  Demux : Demux
  Product{,1..3} (4 alike) : Product  OutDataTypeStr=fixdt(1,20,11)
  Subtract{4..7} (4 alike) : Sum  Inputs=+-  OutDataTypeStr=fixdt(1,20,11)
  Sum of Elements : Sum  Inputs=++++  OutDataTypeStr=fixdt(1,20,11)
  J16 : Outport
  wires:
  Prediction_16/1 -> Demux/1
  Product/1 -> Sum of Elements/1
  iy_ref/1 -> Subtract7/1
  Demux/3 -> Subtract6/2
  Sum of Elements/1 -> J16/1  "J"
  iq_ref/1 -> Subtract5/1
  id_ref/1 -> Subtract4/1
  Demux/2 -> Subtract5/2
  ix_ref/1 -> Subtract6/1
  Demux/4 -> Subtract7/2
  Demux/1 -> Subtract4/2
  Subtract4/1 -> Product/2, Product/1
  Subtract5/1 -> Product1/2, Product1/1
  Product1/1 -> Sum of Elements/2
  Product2/1 -> Sum of Elements/3
  Subtract6/1 -> Product2/1, Product2/2
  Subtract7/1 -> Product3/2, Product3/1
  Product3/1 -> Sum of Elements/4

== system test_cost_function_only_without_delays/HDL_DUT1/Subsystem/Subsystem2 ==
  Prediction_3 : Inport
  id_ref : Inport  Port=2
  iq_ref : Inport  Port=3
  ix_ref : Inport  Port=4
  iy_ref : Inport  Port=5
  Demux : Demux
  Product{1..4} (4 alike) : Product  OutDataTypeStr=fixdt(1,20,11)
  Subtract{4..7} (4 alike) : Sum  Inputs=+-  OutDataTypeStr=fixdt(1,20,11)
  Sum of Elements : Sum  Inputs=++++  OutDataTypeStr=fixdt(1,20,11)
  J3 : Outport
  wires:
  Prediction_3/1 -> Demux/1
  iy_ref/1 -> Subtract7/1
  Demux/3 -> Subtract6/2
  Sum of Elements/1 -> J3/1  "J"
  iq_ref/1 -> Subtract5/1
  id_ref/1 -> Subtract4/1
  Demux/2 -> Subtract5/2
  ix_ref/1 -> Subtract6/1
  Demux/4 -> Subtract7/2
  Demux/1 -> Subtract4/2
  Product3/1 -> Sum of Elements/1
  Product1/1 -> Sum of Elements/2
  Product2/1 -> Sum of Elements/3
  Product4/1 -> Sum of Elements/4
  Subtract4/1 -> Product3/2, Product3/1
  Subtract5/1 -> Product1/2, Product1/1
  Subtract6/1 -> Product2/2, Product2/1
  Subtract7/1 -> Product4/2, Product4/1

== system test_cost_function_only_without_delays/HDL_DUT1/Subsystem/Subsystem3 ==
  Prediction_4 : Inport
  id_ref : Inport  Port=2
  iq_ref : Inport  Port=3
  ix_ref : Inport  Port=4
  iy_ref : Inport  Port=5
  Demux : Demux
  Product{1..4} (4 alike) : Product  OutDataTypeStr=fixdt(1,20,11)
  Subtract{4..7} (4 alike) : Sum  Inputs=+-  OutDataTypeStr=fixdt(1,20,11)
  Sum of Elements : Sum  Inputs=++++  OutDataTypeStr=fixdt(1,20,11)
  J4 : Outport
  wires:
  Prediction_4/1 -> Demux/1
  iy_ref/1 -> Subtract7/1
  Demux/3 -> Subtract6/2
  Sum of Elements/1 -> J4/1  "J"
  iq_ref/1 -> Subtract5/1
  id_ref/1 -> Subtract4/1
  Demux/2 -> Subtract5/2
  ix_ref/1 -> Subtract6/1
  Demux/4 -> Subtract7/2
  Demux/1 -> Subtract4/2
  Product3/1 -> Sum of Elements/1
  Product1/1 -> Sum of Elements/2
  Product2/1 -> Sum of Elements/3
  Product4/1 -> Sum of Elements/4
  Subtract4/1 -> Product3/2, Product3/1
  Subtract5/1 -> Product1/2, Product1/1
  Subtract6/1 -> Product2/2, Product2/1
  Subtract7/1 -> Product4/2, Product4/1

== system test_cost_function_only_without_delays/HDL_DUT1/Subsystem/Subsystem4 ==
  Prediction_5 : Inport
  id_ref : Inport  Port=2
  iq_ref : Inport  Port=3
  ix_ref : Inport  Port=4
  iy_ref : Inport  Port=5
  Demux : Demux
  Product{1..4} (4 alike) : Product  OutDataTypeStr=fixdt(1,20,11)
  Subtract{4..7} (4 alike) : Sum  Inputs=+-  OutDataTypeStr=fixdt(1,20,11)
  Sum of Elements : Sum  Inputs=++++  OutDataTypeStr=fixdt(1,20,11)
  J5 : Outport
  wires:
  Prediction_5/1 -> Demux/1
  iy_ref/1 -> Subtract7/1
  Demux/3 -> Subtract6/2
  Sum of Elements/1 -> J5/1  "J"
  iq_ref/1 -> Subtract5/1
  id_ref/1 -> Subtract4/1
  Demux/2 -> Subtract5/2
  ix_ref/1 -> Subtract6/1
  Demux/4 -> Subtract7/2
  Demux/1 -> Subtract4/2
  Product3/1 -> Sum of Elements/1
  Product1/1 -> Sum of Elements/2
  Product2/1 -> Sum of Elements/3
  Product4/1 -> Sum of Elements/4
  Subtract4/1 -> Product3/1, Product3/2
  Subtract5/1 -> Product1/2, Product1/1
  Subtract6/1 -> Product2/2, Product2/1
  Subtract7/1 -> Product4/2, Product4/1

== system test_cost_function_only_without_delays/HDL_DUT1/Subsystem/Subsystem5 ==
  Prediction_6 : Inport
  id_ref : Inport  Port=2
  iq_ref : Inport  Port=3
  ix_ref : Inport  Port=4
  iy_ref : Inport  Port=5
  Demux : Demux
  Product{1..4} (4 alike) : Product  OutDataTypeStr=fixdt(1,20,11)
  Subtract{4..7} (4 alike) : Sum  Inputs=+-  OutDataTypeStr=fixdt(1,20,11)
  Sum of Elements : Sum  Inputs=++++  OutDataTypeStr=fixdt(1,20,11)
  J6 : Outport
  wires:
  Prediction_6/1 -> Demux/1
  iy_ref/1 -> Subtract7/1
  Demux/3 -> Subtract6/2
  Sum of Elements/1 -> J6/1  "J"
  iq_ref/1 -> Subtract5/1
  id_ref/1 -> Subtract4/1
  Demux/2 -> Subtract5/2
  ix_ref/1 -> Subtract6/1
  Demux/4 -> Subtract7/2
  Demux/1 -> Subtract4/2
  Product3/1 -> Sum of Elements/1
  Product1/1 -> Sum of Elements/2
  Product2/1 -> Sum of Elements/3
  Product4/1 -> Sum of Elements/4
  Subtract4/1 -> Product3/2, Product3/1
  Subtract5/1 -> Product1/1, Product1/2
  Subtract6/1 -> Product2/2, Product2/1
  Subtract7/1 -> Product4/2, Product4/1

== system test_cost_function_only_without_delays/HDL_DUT1/Subsystem/Subsystem6 ==
  Prediction_7 : Inport
  id_ref : Inport  Port=2
  iq_ref : Inport  Port=3
  ix_ref : Inport  Port=4
  iy_ref : Inport  Port=5
  Demux : Demux
  Product{1..4} (4 alike) : Product  OutDataTypeStr=fixdt(1,20,11)
  Subtract{4..7} (4 alike) : Sum  Inputs=+-  OutDataTypeStr=fixdt(1,20,11)
  Sum of Elements : Sum  Inputs=++++  OutDataTypeStr=fixdt(1,20,11)
  J7 : Outport
  wires:
  Prediction_7/1 -> Demux/1
  iy_ref/1 -> Subtract7/1
  Demux/3 -> Subtract6/2
  Sum of Elements/1 -> J7/1  "J"
  iq_ref/1 -> Subtract5/1
  id_ref/1 -> Subtract4/1
  Demux/2 -> Subtract5/2
  ix_ref/1 -> Subtract6/1
  Demux/4 -> Subtract7/2
  Demux/1 -> Subtract4/2
  Product3/1 -> Sum of Elements/1
  Product1/1 -> Sum of Elements/2
  Product2/1 -> Sum of Elements/3
  Product4/1 -> Sum of Elements/4
  Subtract4/1 -> Product3/2, Product3/1
  Subtract5/1 -> Product1/2, Product1/1
  Subtract6/1 -> Product2/2, Product2/1
  Subtract7/1 -> Product4/2, Product4/1

== system test_cost_function_only_without_delays/HDL_DUT1/Subsystem/Subsystem7 ==
  Prediction_8 : Inport
  id_ref : Inport  Port=2
  iq_ref : Inport  Port=3
  ix_ref : Inport  Port=4
  iy_ref : Inport  Port=5
  Demux : Demux
  Product{1..4} (4 alike) : Product  OutDataTypeStr=fixdt(1,20,11)
  Subtract{4..7} (4 alike) : Sum  Inputs=+-  OutDataTypeStr=fixdt(1,20,11)
  Sum of Elements : Sum  Inputs=++++  OutDataTypeStr=fixdt(1,20,11)
  J8 : Outport
  wires:
  Prediction_8/1 -> Demux/1
  iy_ref/1 -> Subtract7/1
  Demux/3 -> Subtract6/2
  Sum of Elements/1 -> J8/1  "J"
  iq_ref/1 -> Subtract5/1
  id_ref/1 -> Subtract4/1
  Demux/2 -> Subtract5/2
  ix_ref/1 -> Subtract6/1
  Demux/4 -> Subtract7/2
  Demux/1 -> Subtract4/2
  Product3/1 -> Sum of Elements/1
  Product1/1 -> Sum of Elements/2
  Product2/1 -> Sum of Elements/3
  Product4/1 -> Sum of Elements/4
  Subtract4/1 -> Product3/1, Product3/2
  Subtract5/1 -> Product1/1, Product1/2
  Subtract6/1 -> Product2/1, Product2/2
  Subtract7/1 -> Product4/2, Product4/1

== system test_cost_function_only_without_delays/HDL_DUT1/Subsystem/Subsystem8 ==
  Prediction_9 : Inport
  id_ref : Inport  Port=2
  iq_ref : Inport  Port=3
  ix_ref : Inport  Port=4
  iy_ref : Inport  Port=5
  Demux : Demux
  Product{1..4} (4 alike) : Product  OutDataTypeStr=fixdt(1,20,11)
  Subtract{4..7} (4 alike) : Sum  Inputs=+-  OutDataTypeStr=fixdt(1,20,11)
  Sum of Elements : Sum  Inputs=++++  OutDataTypeStr=fixdt(1,20,11)
  J9 : Outport
  wires:
  Prediction_9/1 -> Demux/1
  iy_ref/1 -> Subtract7/1
  Demux/3 -> Subtract6/2
  Sum of Elements/1 -> J9/1  "J"
  iq_ref/1 -> Subtract5/1
  id_ref/1 -> Subtract4/1
  Demux/2 -> Subtract5/2
  ix_ref/1 -> Subtract6/1
  Demux/4 -> Subtract7/2
  Demux/1 -> Subtract4/2
  Product3/1 -> Sum of Elements/1
  Product1/1 -> Sum of Elements/2
  Product2/1 -> Sum of Elements/3
  Product4/1 -> Sum of Elements/4
  Subtract4/1 -> Product3/2, Product3/1
  Subtract5/1 -> Product1/2, Product1/1
  Subtract6/1 -> Product2/2, Product2/1
  Subtract7/1 -> Product4/2, Product4/1

== system test_cost_function_only_without_delays/HDL_DUT1/Subsystem/Subsystem9 ==
  Prediction_10 : Inport
  id_ref : Inport  Port=2
  iq_ref : Inport  Port=3
  ix_ref : Inport  Port=4
  iy_ref : Inport  Port=5
  Demux : Demux
  Product{1..4} (4 alike) : Product  OutDataTypeStr=fixdt(1,20,11)
  Subtract{4..7} (4 alike) : Sum  Inputs=+-  OutDataTypeStr=fixdt(1,20,11)
  Sum of Elements : Sum  Inputs=++++  OutDataTypeStr=fixdt(1,20,11)
  J10 : Outport
  wires:
  Prediction_10/1 -> Demux/1
  iy_ref/1 -> Subtract7/1
  Demux/3 -> Subtract6/2
  Sum of Elements/1 -> J10/1  "J"
  iq_ref/1 -> Subtract5/1
  id_ref/1 -> Subtract4/1
  Demux/2 -> Subtract5/2
  ix_ref/1 -> Subtract6/1
  Demux/4 -> Subtract7/2
  Demux/1 -> Subtract4/2
  Product3/1 -> Sum of Elements/1
  Product1/1 -> Sum of Elements/2
  Product2/1 -> Sum of Elements/3
  Product4/1 -> Sum of Elements/4
  Subtract4/1 -> Product3/2, Product3/1
  Subtract5/1 -> Product1/2, Product1/1
  Subtract6/1 -> Product2/2, Product2/1
  Subtract7/1 -> Product4/2, Product4/1
